simulink model "exple_12102017_discrete"  (R2016b)
settings: Solver=VariableStepAuto  StartTime=0.0  StopTime=2  RelTol=1e-3
undefined symbols (not defined in the file): DiscIntNeverNeededParam
settings Model: Creator=live  LastModifiedBy=live

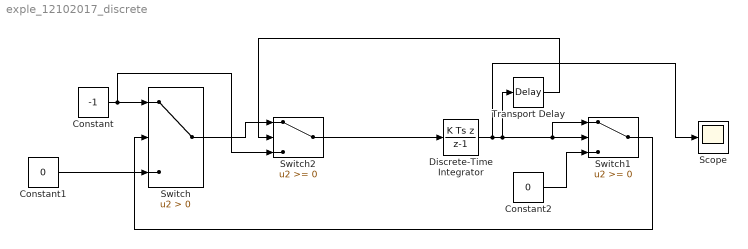
== system exple_12102017_discrete ==
  Constant : Constant  Value=-1
  Constant1 : Constant  Value=0
  Constant2 : Constant  Value=0
  Discrete-Time Integrator : DiscreteIntegrator  IntegratorMethod=Integration: Backward Euler  InitialCondition=1  InitialConditionSetting=State (most efficient)  SampleTime=0.02  ICPrevOutput=DiscIntNeverNeededParam  ICPrevScaledInput=DiscIntNeverNeededParam
  Scope : Scope
  Switch : Switch  Criteria=u2 > Threshold
  Switch1 : Switch
  Switch2 : Switch
  Transport Delay : TransportDelay  DelayTime=0.2  InitialOutput=1
  wires:
  Constant1/1 -> Switch/3
  Discrete-Time Integrator/1 -> Scope/1, Transport Delay/1, Switch1/1, Switch1/2
  Constant2/1 -> Switch1/3
  Constant/1 -> Switch2/3, Switch/1
  Switch1/1 -> Switch/2
  Transport Delay/1 -> Switch2/2
  Switch/1 -> Switch2/1
  Switch2/1 -> Discrete-Time Integrator/1
